simulink model "PassengerCar"  (R2019b)
settings: Solver=ode1  StartTime=0  StopTime=25  FixedStep=1.0000000000000000e-003  RelTol=1e-3
InitFcn:
  | sampleTime = str2double(get_param(bdroot, 'FixedStep'));
undefined symbols (not defined in the file or in its folder): AccPedalPos, BrakePedalPos, BrakeSwitch, DiscIntNeverNeededParam, DYNA4, EngSpd, IgnitionSwitch, InitialGear, InitialSpeed, IntendedEngTrq, LeftIndicator, MainBrakePress, MaxGear, MDL, MinGear, RefAcc, RefLane, RefLatPos, RefPath, RefPathCurv, RefSpd, RefSpdPreview, RefSpdRetrospect, RightIndicator, SteeringWheelAng, SteeringWheelTrq, UserDefinedRefValue, vm_const
libraries: UtilitiesLibrary x31, simulink x18, WheelSystemModules x13, LongitudinalControllerModules x13, LateralControllerModules x7, AnimationBusselectorModules x5, EnvironmentModules x5, BasicEngineControlModules x5, MiscellaneousControlModules x5, Animation3Modules x4, AuxiliariesModules x4, TireModules x4
(part 24 of 39)

== system PassengerCar/Vehicle/WheelSystem/RearLeftWheelSystem/Tire ==
  fromCTRL : Inport
  fromChassis : Inport  Port=2
  fromWheel : Inport  Port=3
  Demux1 : Demux  Outputs=[1 1 1 1 1 1 1]
  Demux2 : Demux  Outputs=[1 1 1 1 1]
  Demux3 : Demux  Outputs=[1 1 1 1 1 1 1]
  Demux4 : Demux  Outputs=[1 1 1]
  Demux5 : Demux  Outputs=[1 1 1]
  DynaComponentInfo : Subsystem  Tag=DynaComponentInfo
      mask init:
      | data= get_param(gcb, 'UserData');
      settings: OpenFcn=DYNA4.ModelHandling.Component.ShowEditComponentInformationDialog(gcb);
      mask Display: disp(['Type = ', data.type, '\nGroup = ', data.group, '\nName = ', data.name])
  InputFromCTRL : Subsystem  Tag=TESIS DYNAware Interface Block  mask{NeedsUpdate=off, SignalInfo=|}
      mask SignalInfo=|
      | {
      |   "Version": "4.6",
      |   "MuxedOutputBusName": "output",
      |   "MuxedInputBusName": "fromCTRL",
      |   "MuxedInputSelected": true,
      |   "MuxedOutputSelected": false,
      |   "SignalData": [
      |     {
      |       "initialValue": "0.0",
      |       "name": "AddRoadElev[m]",
      |       "comment": "",
      |       "minString": "",
      |       "maxString": "",
      |       "width": 1,
      |       "dataType": 0,
      |       "signalType": 0,
      |       "createSignal": false,
      |       "outputName": "AddRoadElev[m]",
      |       "generateSignalAccessBlock": false,
      |       "accessId": "$(parentId).$(blockName).$(outputName)"
      |     },
      |     {
      |       "initialValue": "0.0",
      |       "name": "RoadFrictionScaling[0_2]",
      |       "comment": "",
      |       "minString": "",
      |       "maxString": "",
      |       "width": 1,
      |       "dataType": 0,
      |       "signalType": 0,
      |       "createSignal": false,
      |       "outputName": "RoadFrictionScaling[0_2]",
      |       "generateSignalAccessBlock": false,
      |       "accessId": "$(parentId).$(blockName).$(outputName)"
      |     },
      |     {
      |       "initialValue": "0.0",
      |       "name": "AddLongRoadSlope[-]",
      |       "comment": "",
      |       "minString": "",
      |       "maxString": "",
      |       "width": 1,
      |       "dataType": 0,
      |       "signalType": 0,
      |       "createSignal": false,
      |       "outputName": "AddLongRoadSlope[-]",
      |       "generateSignalAccessBlock": false,
      |       "accessId": "$(parentId).$(blockName).$(outputName)"
      |     },
      |     {
      |       "initialValue": "0.0",
      |       "name": "AddLatRoadSlope[-]",
      |       "comment": "",
      |       "minString": "",
      |       "maxString": "",
      |       "width": 1,
      |       "dataType": 0,
      |       "signalType": 0,
      |       "createSignal": false,
      |       "outputName": "AddLatRoadSlope[-]",
      |       "generateSignalAccessBlock": false,
      |       "accessId": "$(parentId).$(blockName).$(outputName)"
      |     },
      |     {
      |       "initialValue": "0.0",
      |       "name": "LocalRoadSysSwitch[0;1]",
      |       "comment": "",
      |       "minString": "",
      |       "maxString": "",
      |       "width": 1,
      |       "dataType": 0,
      |       "signalType": 0,
      |       "createSignal": false,
      |       "outputName": "LocalRoadSysSwitch[0;1]",
      |       "generateSignalAccessBlock": false,
      |       "accessId": "$(parentId).$(blockName).$(outputName)"
      |     },
      |     {
      |       "initialValue": "0.0",
      |       "name": "RelInflPress[Pa]",
      |       "comment": "",
      |       "minString": "",
      |       "maxString": "",
      |       "width": -1,
      |       "dataType": 0,
      |       "signalType": 0,
      |       "createSignal": false,
      |       "outputName": "RelInflPress[Pa]",
      |       "generateSignalAccessBlock": false,
      |       "accessId": "$(parentId).$(blockName).$(outputName)"
      |     }
      |   ]
      | }
      mask prompts: NeedsUpdate "Specify, if subsystem content needs to be updated"; SignalInfo "Signal Info (json)"
      mask help: DYNA4 Interface Block Version 4.6
      mask init:
      | blockName = get_param(gcbh, 'Name');
      | parentId = DYNA4.ModelHandling.AccessID.getFromHierarchy(gcbh);
      | TD.InterfaceBlock.ModelCallbacks.GenerateContent(gcb);
      settings: DeleteFcn=TD.InterfaceBlock.ModelCallbacks.CloseGUI( gcbh );  NameChangeFcn=TD.InterfaceBlock.ModelCallbacks.BlockRenamedHandler(gcbh);  OpenFcn=TD.InterfaceBlock.ModelCallbacks.OpenGUI( gcbh );  CloseFcn=TD.InterfaceBlock.ModelCallbacks.CloseGUI( gcbh );
      mask Display:
      | image('InterfaceBlock.png','center');
      | port_label('input',1, 'fromCTRL');
      | port_label('output',1, 'AddRoadElev[m]');
      | port_label('output',2, 'RoadFrictionScaling[0_2]');
      | port_label('output',3, 'AddLongRoadSlope[-]');
      | port_label('output',4, 'AddLatRoadSlope[-]');
      | port_label('output',5, 'LocalRoadSysSwitch[0;1]');
      | port_label('output',6, 'RelInflPress[Pa]');
  InputFromChassis : Subsystem  Tag=TESIS DYNAware Interface Block  mask{NeedsUpdate=off, SignalInfo=|}
      mask SignalInfo=|
      | {
      |   "Version": "4.6",
      |   "MuxedOutputBusName": "output",
      |   "MuxedInputBusName": "fromChassis",
      |   "MuxedInputSelected": true,
      |   "MuxedOutputSelected": false,
      |   "SignalData": [
      |     {
      |       "initialValue": "0.0",
      |       "name": "VehicleBody.Pos(WorldSys)[m]",
      |       "comment": "",
      |       "minString": "",
      |       "maxString": "",
      |       "width": 3,
      |       "dataType": 0,
      |       "signalType": 0,
      |       "createSignal": false,
      |       "outputName": "Pos(WorldSys)[m]",
      |       "generateSignalAccessBlock": false,
      |       "accessId": "$(parentId).$(blockName).$(outputName)"
      |     },
      |     {
      |       "initialValue": "0.0",
      |       "name": "VehicleBody.RotMatrix(WorldSys)[-]",
      |       "comment": "",
      |       "minString": "",
      |       "maxString": "",
      |       "width": 9,
      |       "dataType": 0,
      |       "signalType": 0,
      |       "createSignal": false,
      |       "outputName": "RotMatrix(WorldSys)[-]",
      |       "generateSignalAccessBlock": false,
      |       "accessId": "$(parentId).$(blockName).$(outputName)"
      |     },
      |     {
      |       "initialValue": "0.0",
      |       "name": "WheelSystem.WheelRotAxis(VehSys)[-]",
      |       "comment": "",
      |       "minString": "",
      |       "maxString": "",
      |       "width": 3,
      |       "dataType": 0,
      |       "signalType": 0,
      |       "createSignal": false,
      |       "outputName": "WheelRotAxis(VehSys)[-]",
      |       "generateSignalAccessBlock": false,
      |       "accessId": "$(parentId).$(blockName).$(outputName)"
      |     },
      |     {
      |       "initialValue": "0.0",
      |       "name": "WheelSystem.TirePos(VehSys)[m]",
      |       "comment": "",
      |       "minString": "",
      |       "maxString": "",
      |       "width": 3,
      |       "dataType": 0,
      |       "signalType": 0,
      |       "createSignal": false,
      |       "outputName": "TirePos(VehSys)[m]",
      |       "generateSignalAccessBlock": false,
      |       "accessId": "$(parentId).$(blockName).$(outputName)"
      |     },
      |     {
      |       "initialValue": "0.0",
      |       "name": "WheelSystem.TireVel_wrt_WorldSys(VehSys)[m/s]",
      |       "comment": "",
      |       "minString": "",
      |       "maxString": "",
      |       "width": 3,
      |       "dataType": 0,
      |       "signalType": 0,
      |       "createSignal": false,
      |       "outputName": "TireVel_wrt_WorldSys(VehSys)[m/s]",
      |       "generateSignalAccessBlock": false,
      |       "accessId": "$(parentId).$(blockName).$(outputName)"
      |     },
      |     {
      |       "initialValue": "0.0",
      |       "name": "WheelSystem.WheelRotVel_wrt_WorldSys(VehSys)[rad/s]",
      |       "comment": "",
      |       "minString": "",
      |       "maxString": "",
      |       "width": 3,
      |       "dataType": 0,
      |       "signalType": 0,
      |       "createSignal": false,
      |       "outputName": "WheelRotVel_wrt_WorldSys(VehSys)[rad/s]",
      |       "generateSignalAccessBlock": false,
      |       "accessId": "$(parentId).$(blockName).$(outputName)"
      |     }
      |   ]
      | }
      mask prompts: NeedsUpdate "Specify, if subsystem content needs to be updated"; SignalInfo "Signal Info (json)"
      mask help: DYNA4 Interface Block Version 4.6
      mask init:
      | blockName = get_param(gcbh, 'Name');
      | parentId = DYNA4.ModelHandling.AccessID.getFromHierarchy(gcbh);
      | TD.InterfaceBlock.ModelCallbacks.GenerateContent(gcb);
      settings: DeleteFcn=TD.InterfaceBlock.ModelCallbacks.CloseGUI( gcbh );  NameChangeFcn=TD.InterfaceBlock.ModelCallbacks.BlockRenamedHandler(gcbh);  OpenFcn=TD.InterfaceBlock.ModelCallbacks.OpenGUI( gcbh );  CloseFcn=TD.InterfaceBlock.ModelCallbacks.CloseGUI( gcbh );
      mask Display:
      | image('InterfaceBlock.png','center');
      | port_label('input',1, 'fromChassis');
      | port_label('output',1, 'Pos(WorldSys)[m]');
      | port_label('output',2, 'RotMatrix(WorldSys)[-]');
      | port_label('output',3, 'WheelRotAxis(VehSys)[-]');
      | port_label('output',4, 'TirePos(VehSys)[m]');
      | port_label('output',5, 'TireVel_wrt_WorldSys(VehSys)[m/s]');
      | port_label('output',6, 'WheelRotVel_wrt_WorldSys(VehSys)[rad/s]');
  InputFromWheel : Subsystem  Tag=TESIS DYNAware Interface Block  mask{NeedsUpdate=off, SignalInfo=|}
      mask SignalInfo=|
      | {
      |   "Version": "4.6",
      |   "MuxedOutputBusName": "fromWheel",
      |   "MuxedInputBusName": "fromWheel",
      |   "MuxedInputSelected": true,
      |   "MuxedOutputSelected": false,
      |   "SignalData": {
      |     "initialValue": "0.0",
      |     "name": "RotSpd[rad/s]",
      |     "comment": "",
      |     "minString": "",
      |     "maxString": "",
      |     "width": 1,
      |     "dataType": 0,
      |     "signalType": 0,
      |     "createSignal": false,
      |     "outputName": "RotSpd[rad/s]",
      |     "generateSignalAccessBlock": false,
      |     "accessId": "$(parentId).$(blockName).$(outputName)"
      |   }
      | }
      mask prompts: NeedsUpdate "Specify, if subsystem content needs to be updated"; SignalInfo "Signal Info (json)"
      mask help: DYNA4 Interface Block Version 4.6
      mask init:
      | blockName = get_param(gcbh, 'Name');
      | parentId = DYNA4.ModelHandling.AccessID.getFromHierarchy(gcbh);
      | TD.InterfaceBlock.ModelCallbacks.GenerateContent(gcb);
      settings: DeleteFcn=TD.InterfaceBlock.ModelCallbacks.CloseGUI( gcbh );  NameChangeFcn=TD.InterfaceBlock.ModelCallbacks.BlockRenamedHandler(gcbh);  OpenFcn=TD.InterfaceBlock.ModelCallbacks.OpenGUI( gcbh );  CloseFcn=TD.InterfaceBlock.ModelCallbacks.CloseGUI( gcbh );
      mask Display:
      | image('InterfaceBlock.png','center');
      | port_label('input',1, 'fromWheel');
      | port_label('output',1, 'RotSpd[rad/s]');
  TMEasy5 : TireModules/TMEasy5  DATA_NODE=MDL.Vehicle.WheelSystem.RearLeft.Tire.TMEasy5  Enable=MDL.Vehicle.WheelSystem.RearLeft.Tire.TMEasy5.Enable  GeneralConstants=MDL.Vehicle.WheelSystem.RearLeft.Tire.TMEasy5.GeneralConstants  ParameterConstants=MDL.Vehicle.WheelSystem.RearLeft.Tire.TMEasy5.ParameterConstants  AdvancedOptions=MDL.Vehicle.WheelSystem.RearLeft.Tire.TMEasy5.AdvancedOptions  sample_time=-1
  TireOutput : Subsystem  Tag=TESIS DYNAware Interface Block  mask{NeedsUpdate=off, SignalInfo=|}
      mask SignalInfo=|
      | {
      |   "Version": "4.6",
      |   "MuxedOutputBusName": "Tire",
      |   "MuxedInputBusName": "input",
      |   "MuxedInputSelected": false,
      |   "MuxedOutputSelected": true,
      |   "SignalData": [
      |     {
      |       "initialValue": "0.0",
      |       "name": "ContactPointPos_wrt_WheelCenter(WorldSys)[m]",
      |       "comment": "",
      |       "minString": "",
      |       "maxString": "",
      |       "width": 3,
      |       "dataType": 0,
      |       "signalType": 0,
      |       "createSignal": false,
      |       "outputName": "ContactPointPos_wrt_WheelCenter(WorldSys)[m]",
      |       "generateSignalAccessBlock": false,
      |       "accessId": "$(parentId).$(blockName).$(outputName)"
      |     },
      |     {
      |       "initialValue": "0.0",
      |       "name": "CamberAng(ContactSys)[rad]",
      |       "comment": "",
      |       "minString": "",
      |       "maxString": "",
      |       "width": 1,
      |       "dataType": 0,
      |       "signalType": 0,
      |       "createSignal": false,
      |       "outputName": "CamberAng(ContactSys)[rad]",
      |       "generateSignalAccessBlock": false,
      |       "accessId": "$(parentId).$(blockName).$(outputName)"
      |     },
      |     {
      |       "initialValue": "0.0",
      |       "name": "TireDefl[m]",
      |       "comment": "",
      |       "minString": "",
      |       "maxString": "",
      |       "width": 1,
      |       "dataType": 0,
      |       "signalType": 0,
      |       "createSignal": false,
      |       "outputName": "TireDefl[m]",
      |       "generateSignalAccessBlock": false,
      |       "accessId": "$(parentId).$(blockName).$(outputName)"
      |     },
      |     {
      |       "initialValue": "0.0",
      |       "name": "TireDeflSpd[m/s]",
      |       "comment": "",
      |       "minString": "",
      |       "maxString": "",
      |       "width": 1,
      |       "dataType": 0,
      |       "signalType": 0,
      |       "createSignal": false,
      |       "outputName": "TireDeflSpd[m/s]",
      |       "generateSignalAccessBlock": false,
      |       "accessId": "$(parentId).$(blockName).$(outputName)"
      |     },
      |     {
      |       "initialValue": "0.0",
      |       "name": "LongSpd(ContactSys)[m/s]",
      |       "comment": "",
      |       "minString": "",
      |       "maxString": "",
      |       "width": 1,
      |       "dataType": 0,
      |       "signalType": 0,
      |       "createSignal": false,
      |       "outputName": "LongSpd(ContactSys)[m/s]",
      |       "generateSignalAccessBlock": false,
      |       "accessId": "$(parentId).$(blockName).$(outputName)"
      |     },
      |     {
      |       "initialValue": "0.0",
      |       "name": "LatSpd(ContactSys)[m/s]",
      |       "comment": "",
      |       "minString": "",
      |       "maxString": "",
      |       "width": 1,
      |       "dataType": 0,
      |       "signalType": 0,
      |       "createSignal": false,
      |       "outputName": "LatSpd(ContactSys)[m/s]",
      |       "generateSignalAccessBlock": false,
      |       "accessId": "$(parentId).$(blockName).$(outputName)"
      |     },
      |     {
      |       "initialValue": "0.0",
      |       "name": "BoreSpd(ContactSys)[rad/s]",
      |       "comment": "",
      |       "minString": "",
      |       "maxString": "",
      |       "width": 1,
      |       "dataType": 0,
      |       "signalType": 0,
      |       "createSignal": false,
      |       "outputName": "BoreSpd(ContactSys)[rad/s]",
      |       "generateSignalAccessBlock": false,
      |       "accessId": "$(parentId).$(blockName).$(outputName)"
      |     },
      |     {
      |       "initialValue": "0.0",
      |       "name": "LongFrcLeverArm_wrt_WheelRotAxis[m]",
      |       "comment": "",
      |       "minString": "",
      |       "maxString": "",
      |       "width": 1,
      |       "dataType": 0,
      |       "signalType": 0,
      |       "createSignal": false,
      |       "outputName": "LongFrcLeverArm_wrt_WheelRotAxis[m]",
      |       "generateSignalAccessBlock": false,
      |       "accessId": "$(parentId).$(blockName).$(outputName)"
      |     },
      |     {
      |       "initialValue": "0.0",
      |       "name": "LongUnitVector(WorldSys)[-]",
      |       "comment": "",
      |       "minString": "",
      |       "maxString": "",
      |       "width": 3,
      |       "dataType": 0,
      |       "signalType": 0,
      |       "createSignal": false,
      |       "outputName": "LongUnitVector(WorldSys)[-]",
      |       "generateSignalAccessBlock": false,
      |       "accessId": "$(parentId).$(blockName).$(outputName)"
      |     },
      |     {
      |       "initialValue": "0.0",
      |       "name": "LatUnitVector(WorldSys)[-]",
      |       "comment": "",
      |       "minString": "",
      |       "maxString": "",
      |       "width": 3,
      |       "dataType": 0,
      |       "signalType": 0,
      |       "createSignal": false,
      |       "outputName": "LatUnitVector(WorldSys)[-]",
      |       "generateSignalAccessBlock": false,
      |       "accessId": "$(parentId).$(blockName).$(outputName)"
      |     },
      |     {
      |       "initialValue": "0.0",
      |       "name": "RoadNormalVector(WorldSys)[-]",
      |       "comment": "",
      |       "minString": "",
      |       "maxString": "",
      |       "width": 3,
      |       "dataType": 0,
      |       "signalType": 0,
      |       "createSignal": false,
      |       "outputName": "RoadNormalVector(WorldSys)[-]",
      |       "generateSignalAccessBlock": false,
      |       "accessId": "$(parentId).$(blockName).$(outputName)"
      |     },
      |     {
      |       "initialValue": "0.0",
      |       "name": "RoadType[-]",
      |       "comment": "",
      |       "minString": "",
      |       "maxString": "",
      |       "width": 1,
      |       "dataType": 0,
      |       "signalType": 0,
      |       "createSignal": false,
      |       "outputName": "RoadType[-]",
      |       "generateSignalAccessBlock": false,
      |       "accessId": "$(parentId).$(blockName).$(outputName)"
      |     },
      |     {
      |       "initialValue": "0.0",
      |       "name": "RoadFrictionScalingCoeff[-]",
      |       "comment": "",
      |       "minString": "",
      |       "maxString": "",
      |       "width": 1,
      |       "dataType": 0,
      |       "signalType": 0,
      |       "createSignal": false,
      |       "outputName": "RoadFrictionScalingCoeff[-]",
      |       "generateSignalAccessBlock": false,
      |       "accessId": "$(parentId).$(blockName).$(outputName)"
      |     },
      |     {
      |       "initialValue": "0.0",
      |       "name": "ContactPointPos(WorldSys)[m]",
      |       "comment": "",
      |       "minString": "",
      |       "maxString": "",
      |       "width": 3,
      |       "dataType": 0,
      |       "signalType": 0,
      |       "createSignal": false,
      |       "outputName": "ContactPointPos(WorldSys)[m]",
      |       "generateSignalAccessBlock": false,
      |       "accessId": "$(parentId).$(blockName).$(outputName)"
      |     },
      |     {
      |       "initialValue": "0.0",
      |       "name": "WheelCenterFrc(VehSys)[N]",
      |       "comment": "",
      |       "minString": "",
      |       "maxString": "",
      |       "width": 3,
      |       "dataType": 0,
      |       "signalType": 0,
      |       "createSignal": false,
      |       "outputName": "WheelCenterFrc(VehSys)[N]",
      |       "generateSignalAccessBlock": false,
      |       "accessId": "$(parentId).$(blockName).$(outputName)"
      |     },
      |     {
      |       "initialValue": "0.0",
      |       "name": "WheelCenterTrq(VehSys)[Nm]",
      |       "comment": "",
      |       "minString": "",
      |       "maxString": "",
      |       "width": 3,
      |       "dataType": 0,
      |       "signalType": 0,
      |       "createSignal": false,
      |       "outputName": "WheelCenterTrq(VehSys)[Nm]",
      |       "generateSignalAccessBlock": false,
      |       "accessId": "$(parentId).$(blockName).$(outputName)"
      |     },
      |     {
      |       "initialValue": "0.0",
      |       "name": "CircumferentialTrq_wrt_WheelRotAxis[Nm]",
      |       "comment": "",
      |       "minString": "",
      |       "maxString": "",
      |       "width": 1,
      |       "dataType": 0,
      |       "signalType": 0,
      |       "createSignal": false,
      |       "outputName": "CircumferentialTrq_wrt_WheelRotAxis[Nm]",
      |       "generateSignalAccessBlock": false,
      |       "accessId": "$(parentId).$(blockName).$(outputName)"
      |     },
      |     {
      |       "initialValue": "0.0",
      |       "name": "MaxRollResistTrq[Nm]",
      |       "comment": "",
      |       "minString": "",
      |       "maxString": "",
      |       "width": 1,
      |       "dataType": 0,
      |       "signalType": 0,
      |       "createSignal": false,
      |       "outputName": "MaxRollResistTrq[Nm]",
      |       "generateSignalAccessBlock": false,
      |       "accessId": "$(parentId).$(blockName).$(outputName)"
      |     },
      |     {
      |       "initialValue": "0.0",
      |       "name": "LatDefl(ContactSys)[m]",
      |       "comment": "",
      |       "minString": "",
      |       "maxString": "",
      |       "width": 1,
      |       "dataType": 0,
      |       "signalType": 0,
      |       "createSignal": false,
      |       "outputName": "LatDefl(ContactSys)[m]",
      |       "generateSignalAccessBlock": false,
      |       "accessId": "$(parentId).$(blockName).$(outputName)"
      |     },
      |     {
      |       "initialValue": "0.0",
      |       "name": "VertStiff[N/m]",
      |       "comment": "",
      |       "minString": "",
      |       "maxString": "",
      |       "width": 1,
      |       "dataType": 0,
      |       "signalType": 0,
      |       "createSignal": false,
      |       "outputName": "VertStiff[N/m]",
      |       "generateSignalAccessBlock": false,
      |       "accessId": "$(parentId).$(blockName).$(outputName)"
      |     },
      |     {
      |       "initialValue": "0.0",
      |       "name": "UnloadedRadius[m]",
      |       "comment": "",
      |       "minString": "",
      |       "maxString": "",
      |       "width": 1,
      |       "dataType": 0,
      |       "signalType": 0,
      |       "createSignal": false,
      |       "outputName": "UnloadedRadius[m]",
      |       "generateSignalAccessBlock": false,
      |       "accessId": "$(parentId).$(blockName).$(outputName)"
      |     },
      |     {
      |       "initialValue": "0.0",
      |       "name": "RimRadius[m]",
      |       "comment": "",
      |       "minString": "",
      |       "maxString": "",
      |       "width": 1,
      |       "dataType": 0,
      |       "signalType": 0,
      |       "createSignal": false,
      |       "outputName": "RimRadius[m]",
      |       "generateSignalAccessBlock": false,
      |       "accessId": "$(parentId).$(blockName).$(outputName)"
      |     },
      |     {
      |       "initialValue": "0.0",
      |       "name": "Width[m]",
      |       "comment": "",
      |       "minString": "",
      |       "maxString": "",
      |       "width": 1,
      |       "dataType": 0,
      |       "signalType": 0,
      |       "createSignal": false,
      |       "outputName": "Width[m]",
      |       "generateSignalAccessBlock": false,
      |       "accessId": "$(parentId).$(blockName).$(outputName)"
      |     },
      |     {
      |       "initialValue": "0.0",
      |       "name": "ContactPointFrc(ContactSys)[N]",
      |       "comment": "",
      |       "minString": "",
      |       "maxString": "",
      |       "width": 3,
      |       "dataType": 0,
      |       "signalType": 0,
      |       "createSignal": false,
      |       "outputName": "ContactPointFrc(ContactSys)[N]",
      |       "generateSignalAccessBlock": false,
      |       "accessId": "$(parentId).$(blockName).$(outputName)"
      |     },
      |     {
      |       "initialValue": "0.0",
      |       "name": "CorneringStiff[N]",
      |       "comment": "",
      |       "minString": "",
      |       "maxString": "",
      |       "width": 1,
      |       "dataType": 0,
      |       "signalType": 0,
      |       "createSignal": false,
      |       "outputName": "CorneringStiff[N]",
      |       "generateSignalAccessBlock": false,
      |       "accessId": "$(parentId).$(blockName).$(outputName)"
      |     },
      |     {
      |       "initialValue": "0.0",
      |       "name": "DynamicRadius[m]",
      |       "comment": "",
      |       "minString": "",
      |       "maxString": "",
      |       "width": 1,
      |       "dataType": 0,
      |       "signalType": 0,
      |       "createSignal": false,
      |       "outputName": "DynamicRadius[m]",
      |       "generateSignalAccessBlock": false,
      |       "accessId": "$(parentId).$(blockName).$(outputName)"
      |     },
      |     {
      |       "initialValue": "0.0",
      |       "name": "Stabilization.DerivativeOfLongFrc_wrt_LongSpd(ContactSys)[N/(m/s)]",
      |       "comment": "",
      |       "minString": "",
      |       "maxString": "",
      |       "width": 1,
      |       "dataType": 0,
      |       "signalType": 0,
      |       "createSignal": false,
      |       "outputName": "Stabilization.DerivativeOfLongFrc_wrt_LongSpd(ContactSys)[N/(m/s)]",
      |       "generateSignalAccessBlock": false,
      |       "accessId": "$(parentId).$(blockName).$(outputName)"
      |     },
      |     {
      |       "initialValue": "0.0",
      |       "name": "Stabilization.DerivativeOfLongTrq_wrt_LongSpd(ContactSys)[Nm/(m/s)]",
      |       "comment": "",
      |       "minString": "",
      |       "maxString": "",
      |       "width": 1,
      |       "dataType": 0,
      |       "signalType": 0,
      |       "createSignal": false,
      |       "outputName": "Stabilization.DerivativeOfLongTrq_wrt_LongSpd(ContactSys)[Nm/(m/s)]",
      |       "generateSignalAccessBlock": false,
      |       "accessId": "$(parentId).$(blockName).$(outputName)"
      |     },
      |     {
      |       "initialValue": "0.0",
      |       "name": "Stabilization.DerivativeOfLatFrc_wrt_LatSpd(ContactSys)[N/(m/s)]",
      |       "comment": "",
      |       "minString": "",
      |       "maxString": "",
      |       "width": 1,
      |       "dataType": 0,
      |       "signalType": 0,
      |       "createSignal": false,
      |       "outputName": "Stabilization.DerivativeOfLatFrc_wrt_LatSpd(ContactSys)[N/(m/s)]",
      |       "generateSignalAccessBlock": false,
      |       "accessId": "$(parentId).$(blockName).$(outputName)"
      |     },
      |     {
      |       "initialValue": "0.0",
      |       "name": "Stabilization.DerivativeOfLatTrq_wrt_LatSpd(ContactSys)[Nm/(m/s)]",
      |       "comment": "",
      |       "minString": "",
      |       "maxString": "",
      |       "width": 1,
      |       "dataType": 0,
      |       "signalType": 0,
      |       "createSignal": false,
      |       "outputName": "Stabilization.DerivativeOfLatTrq_wrt_LatSpd(ContactSys)[Nm/(m/s)]",
      |       "generateSignalAccessBlock": false,
      |       "accessId": "$(parentId).$(blockName).$(outputName)"
      |     },
      |     {
      |       "initialValue": "0.0",
      |       "name": "Stabilization.DerivativeOfBoreTrq_wrt_BoreSpd(ContactSys)[Nm/(rad/s)]",
      |       "comment": "",
      |       "minString": "",
      |       "maxString": "",
      |       "width": 1,
      |       "dataType": 0,
      |       "signalType": 0,
      |       "createSignal": false,
      |       "outputName": "Stabilization.DerivativeOfBoreTrq_wrt_BoreSpd(ContactSys)[Nm/(rad/s)]",
      |       "generateSignalAccessBlock": false,
      |       "accessId": "$(parentId).$(blockName).$(outputName)"
      |     },
      |     {
      |       "initialValue": "0.0",
      |       "name": "SelfAligningTrq[Nm]",
      |       "comment": "",
      |       "minString": "",
      |       "maxString": "",
      |       "width": 1,
      |       "dataType": 0,
      |       "signalType": 0,
      |       "createSignal": false,
      |       "outputName": "SelfAligningTrq[Nm]",
      |       "generateSignalAccessBlock": false,
      |       "accessId": "$(parentId).$(blockName).$(outputName)"
      |     },
      |     {
      |       "initialValue": "0.0",
      |       "name": "RollResistTrq[Nm]",
      |       "comment": "",
      |       "minString": "",
      |       "maxString": "",
      |       "width": 1,
      |       "dataType": 0,
      |       "signalType": 0,
      |       "createSignal": false,
      |       "outputName": "RollResistTrq[Nm]",
      |       "generateSignalAccessBlock": false,
      |       "accessId": "$(parentId).$(blockName).$(outputName)"
      |     },
      |     {
      |       "initialValue": "0.0",
      |       "name": "TippingTrq[Nm]",
      |       "comment": "",
      |       "minString": "",
      |       "maxString": "",
      |       "width": 1,
      |       "dataType": 0,
      |       "signalType": 0,
      |       "createSignal": false,
      |       "outputName": "TippingTrq[Nm]",
      |       "generateSignalAccessBlock": false,
      |       "accessId": "$(parentId).$(blockName).$(outputName)"
      |     },
      |     {
      |       "initialValue": "0.0",
      |       "name": "BoreTrq[Nm]",
      |       "comment": "",
      |       "minString": "",
      |       "maxString": "",
      |       "width": 1,
      |       "dataType": 0,
      |       "signalType": 0,
      |       "createSignal": false,
      |       "outputName": "BoreTrq[Nm]",
      |       "generateSignalAccessBlock": false,
      |       "accessId": "$(parentId).$(blockName).$(outputName)"
      |     },
      |     {
      |       "initialValue": "0.0",
      |       "name": "NormalizedLongSlip[-]",
      |       "comment": "",
      |       "minString": "",
      |       "maxString": "",
      |       "width": 1,
      |       "dataType": 0,
      |       "signalType": 0,
      |       "createSignal": false,
      |       "outputName": "NormalizedLongSlip[-]",
      |       "generateSignalAccessBlock": false,
      |       "accessId": "$(parentId).$(blockName).$(outputName)"
      |     },
      |     {
      |       "initialValue": "0.0",
      |       "name": "NormalizedLatSlip[-]",
      |       "comment": "",
      |       "minString": "",
      |       "maxString": "",
      |       "width": 1,
      |       "dataType": 0,
      |       "signalType": 0,
      |       "createSignal": false,
      |       "outputName": "NormalizedLatSlip[-]",
      |       "generateSignalAccessBlock": false,
      |       "accessId": "$(parentId).$(blockName).$(outputName)"
      |     },
      |     {
      |       "initialValue": "0.0",
      |       "name": "LongSlip[-]",
      |       "comment": "",
      |       "minString": "",
      |       "maxString": "",
      |       "width": 1,
      |       "dataType": 0,
      |       "signalType": 0,
      |       "createSignal": false,
      |       "outputName": "LongSlip[-]",
      |       "generateSignalAccessBlock": false,
      |       "accessId": "$(parentId).$(blockName).$(outputName)"
      |     },
      |     {
      |       "initialValue": "0.0",
      |       "name": "LatSlip[-]",
      |       "comment": "",
      |       "minString": "",
      |       "maxString": "",
      |       "width": 1,
      |       "dataType": 0,
      |       "signalType": 0,
      |       "createSignal": false,
      |       "outputName": "LatSlip[-]",
      |       "generateSignalAccessBlock": false,
      |       "accessId": "$(parentId).$(blockName).$(outputName)"
      |     },
      |     {
      |       "initialValue": "0.0",
      |       "name": "BoreSlip[-]",
      |       "comment": "",
      |       "minString": "",
      |       "maxString": "",
      |       "width": 1,
      |       "dataType": 0,
      |       "signalType": 0,
      |       "createSignal": false,
      |       "outputName": "BoreSlip[-]",
      |       "generateSignalAccessBlock": false,
      |       "accessId": "$(parentId).$(blockName).$(outputName)"
      |     },
      |     {
      |       "initialValue": "0.0",
      |       "name": "CombinedSlip[-]",
      |       "comment": "",
      |       "minString": "",
      |       "maxString": "",
      |       "width": 1,
      |       "dataType": 0,
      |       "signalType": 0,
      |       "createSignal": false,
      |       "outputName": "CombinedSlip[-]",
      |       "generateSignalAccessBlock": false,
      |       "accessId": "$(parentId).$(blockName).$(outputName)"
      |     },
      |     {
      |       "initialValue": "0.0",
      |       "name": "GeneralizedSlip[-]",
      |       "comment": "",
      |       "minString": "",
      |       "maxString": "",
      |       "width": 1,
      |       "dataType": 0,
      |       "signalType": 0,
      |       "createSignal": false,
      |       "outputName": "GeneralizedSlip[-]",
      |       "generateSignalAccessBlock": false,
      |       "accessId": "$(parentId).$(blockName).$(outputName)"
      |     },
      |     {
      |       "initialValue": "0.0",
      |       "name": "GradientOfCombinedFrcAtNoSlip[N/-]",
      |       "comment": "",
      |       "minString": "",
      |       "maxString": "",
      |       "width": 1,
      |       "dataType": 0,
      |       "signalType": 0,
      |       "createSignal": false,
      |       "outputName": "GradientOfCombinedFrcAtNoSlip[N/-]",
      |       "generateSignalAccessBlock": false,
      |       "accessId": "$(parentId).$(blockName).$(outputName)"
      |     },
      |     {
      |       "initialValue": "0.0",
      |       "name": "CombinedMaxFrc[N]",
      |       "comment": "",
      |       "minString": "",
      |       "maxString": "",
      |       "width": 1,
      |       "dataType": 0,
      |       "signalType": 0,
      |       "createSignal": false,
      |       "outputName": "CombinedMaxFrc[N]",
      |       "generateSignalAccessBlock": false,
      |       "accessId": "$(parentId).$(blockName).$(outputName)"
      |     },
      |     {
      |       "initialValue": "0.0",
      |       "name": "CombinedMaxSlipAtCombinedMaxFrc[-]",
      |       "comment": "",
      |       "minString": "",
      |       "maxString": "",
      |       "width": 1,
      |       "dataType": 0,
      |       "signalType": 0,
      |       "createSignal": false,
      |       "outputName": "CombinedMaxSlipAtCombinedMaxFrc[-]",
      |       "generateSignalAccessBlock": false,
      |       "accessId": "$(parentId).$(blockName).$(outputName)"
      |     },
      |     {
      |       "initialValue": "0.0",
      |       "name": "CombinedSlideFrc[N]",
      |       "comment": "",
      |       "minString": "",
      |       "maxString": "",
      |       "width": 1,
      |       "dataType": 0,
      |       "signalType": 0,
      |       "createSignal": false,
      |       "outputName": "CombinedSlideFrc[N]",
      |       "generateSignalAccessBlock": false,
      |       "accessId": "$(parentId).$(blockName).$(outputName)"
      |     },
      |     {
      |       "initialValue": "0.0",
      |       "name": "CombinedSlipAtCombinedSlideFrc[-]",
      |       "comment": "",
      |       "minString": "",
      |       "maxString": "",
      |       "width": 1,
      |       "dataType": 0,
      |       "signalType": 0,
      |       "createSignal": false,
      |       "outputName": "CombinedSlipAtCombinedSlideFrc[-]",
      |       "generateSignalAccessBlock": false,
      |       "accessId": "$(parentId).$(blockName).$(outputName)"
      |     },
      |     {
      |       "initialValue": "0.0",
      |       "name": "CombinedForce[N]",
      |       "comment": "",
      |       "minString": "",
      |       "maxString": "",
      |       "width": 1,
      |       "dataType": 0,
      |       "signalType": 0,
      |       "createSignal": false,
      |       "outputName": "CombinedForce[N]",
      |       "generateSignalAccessBlock": false,
      |       "accessId": "$(parentId).$(blockName).$(outputName)"
      |     },
      |     {
      |       "initialValue": "0.0",
      |       "name": "DerivativeOfCombinedFrc_wrt_CombinedSlip[N/-]",
      |       "comment": "",
      |       "minString": "",
      |       "maxString": "",
      |       "width": 1,
      |       "dataType": 0,
      |       "signalType": 0,
      |       "createSignal": false,
      |       "outputName": "DerivativeOfCombinedFrc_wrt_CombinedSlip[N/-]",
      |       "generateSignalAccessBlock": false,
      |       "accessId": "$(parentId).$(blockName).$(outputName)"
      |     },
      |     {
      |       "initialValue": "0.0",
      |       "name": "BoreRadius[m]",
      |       "comment": "",
      |       "minString": "",
      |       "maxString": "",
      |       "width": 1,
      |       "dataType": 0,
      |       "signalType": 0,
      |       "createSignal": false,
      |       "outputName": "BoreRadius[m]",
      |       "generateSignalAccessBlock": false,
      |       "accessId": "$(parentId).$(blockName).$(outputName)"
      |     },
      |     {
      |       "initialValue": "0.0",
      |       "name": "TireRotSpd[rad/s]",
      |       "comment": "",
      |       "minString": "",
      |       "maxString": "",
      |       "width": 1,
      |       "dataType": 0,
      |       "signalType": 0,
      |       "createSignal": false,
      |       "outputName": "TireRotSpd[rad/s]",
      |       "generateSignalAccessBlock": false,
      |       "accessId": "$(parentId).$(blockName).$(outputName)"
      |     },
      |     {
      |       "initialValue": "0.0",
      |       "name": "CamberFrc[N]",
      |       "comment": "",
      |       "minString": "",
      |       "maxString": "",
      |       "width": 1,
      |       "dataType": 0,
      |       "signalType": 0,
      |       "createSignal": false,
      |       "outputName": "CamberFrc[N]",
      |       "generateSignalAccessBlock": false,
      |       "accessId": "$(parentId).$(blockName).$(outputName)"
      |     },
      |     {
      |       "initialValue": "0.0",
      |       "name": "LongRelaxationTime[s]",
      |       "comment": "",
      |       "minString": "",
      |       "maxString": "",
      |       "width": 1,
      |       "dataType": 0,
      |       "signalType": 0,
      |       "createSignal": false,
      |       "outputName": "LongRelaxationTime[s]",
      |       "generateSignalAccessBlock": false,
      |       "accessId": "$(parentId).$(blockName).$(outputName)"
      |     },
      |     {
      |       "initialValue": "0.0",
      |       "name": "LatRelaxationTime[s]",
      |       "comment": "",
      |       "minString": "",
      |       "maxString": "",
      |       "width": 1,
      |       "dataType": 0,
      |       "signalType": 0,
      |       "createSignal": false,
      |       "outputName": "LatRelaxationTime[s]",
      |       "generateSignalAccessBlock": false,
      |       "accessId": "$(parentId).$(blockName).$(outputName)"
      |     },
      |     {
      |       "initialValue": "0.0",
      |       "name": "TorsionalRelaxationTime[s]",
      |       "comment": "",
      |       "minString": "",
      |       "maxString": "",
      |       "width": 1,
      |       "dataType": 0,
      |       "signalType": 0,
      |       "createSignal": false,
      |       "outputName": "TorsionalRelaxationTime[s]",
      |       "generateSignalAccessBlock": false,
      |       "accessId": "$(parentId).$(blockName).$(outputName)"
      |     },
      |     {
      |       "initialValue": "0.0",
      |       "name": "LongRelaxationLength[m]",
      |       "comment": "",
      |       "minString": "",
      |       "maxString": "",
      |       "width": 1,
      |       "dataType": 0,
      |       "signalType": 0,
      |       "createSignal": false,
      |       "outputName": "LongRelaxationLength[m]",
      |       "generateSignalAccessBlock": false,
      |       "accessId": "$(parentId).$(blockName).$(outputName)"
      |     },
      |     {
      |       "initialValue": "0.0",
      |       "name": "LatRelaxationLength[m]",
      |       "comment": "",
      |       "minString": "",
      |       "maxString": "",
      |       "width": 1,
      |       "dataType": 0,
      |       "signalType": 0,
      |       "createSignal": false,
      |       "outputName": "LatRelaxationLength[m]",
      |       "generateSignalAccessBlock": false,
      |       "accessId": "$(parentId).$(blockName).$(outputName)"
      |     },
      |     {
      |       "initialValue": "0.0",
      |       "name": "TorsionalRelaxationAngle[rad]",
      |       "comment": "",
      |       "minString": "",
      |       "maxString": "",
      |       "width": 1,
      |       "dataType": 0,
      |       "signalType": 0,
      |       "createSignal": false,
      |       "outputName": "TorsionalRelaxationAngle[rad]",
      |       "generateSignalAccessBlock": false,
      |       "accessId": "$(parentId).$(blockName).$(outputName)"
      |     },
      |     {
      |       "initialValue": "0.0",
      |       "name": "ContactPointTrq(ContactSys)[Nm]",
      |       "comment": "",
      |       "minString": "",
      |       "maxString": "",
      |       "width": 3,
      |       "dataType": 0,
      |       "signalType": 0,
      |       "createSignal": false,
      |       "outputName": "ContactPointTrq(ContactSys)[Nm]",
      |       "generateSignalAccessBlock": false,
      |       "accessId": "$(parentId).$(blockName).$(outputName)"
      |     },
      |     {
      |       "initialValue": "0.0",
      |       "name": "ContactPatchLength[m]",
      |       "comment": "",
      |       "minString": "",
      |       "maxString": "",
      |       "width": 1,
      |       "dataType": 0,
      |       "signalType": 0,
      |       "createSignal": false,
      |       "outputName": "ContactPatchLength[m]",
      |       "generateSignalAccessBlock": false,
      |       "accessId": "$(parentId).$(blockName).$(outputName)"
      |     },
      |     {
      |       "initialValue": "0.0",
      |       "name": "ContactPatchWidth[m]",
      |       "comment": "",
      |       "minString": "",
      |       "maxString": "",
      |       "width": 1,
      |       "dataType": 0,
      |       "signalType": 0,
      |       "createSignal": false,
      |       "outputName": "ContactPatchWidth[m]",
      |       "generateSignalAccessBlock": false,
      |       "accessId": "$(parentId).$(blockName).$(outputName)"
      |     },
      |     {
      |       "initialValue": "0.0",
      |       "name": "LocalContactPoints(WorldSys)[m]",
      |       "comment": "",
      |       "minString": "",
      |       "maxString": "",
      |       "width": 12,
      |       "dataType": 0,
      |       "signalType": 0,
      |       "createSignal": false,
      |       "outputName": "LocalContactPoints(WorldSys)[m]",
      |       "generateSignalAccessBlock": false,
      |       "accessId": "$(parentId).$(blockName).$(outputName)"
      |     },
      |     {
      |       "initialValue": "0.0",
      |       "name": "NumberOfLocalContactPoints[-]",
      |       "comment": "",
      |       "minString": "",
      |       "maxString": "",
      |       "width": 1,
      |       "dataType": 0,
      |       "signalType": 0,
      |       "createSignal": false,
      |       "outputName": "NumberOfLocalContactPoints[-]",
      |       "generateSignalAccessBlock": false,
      |       "accessId": "$(parentId).$(blockName).$(outputName)"
      |     }
      |   ]
      | }
      mask prompts: NeedsUpdate "Specify, if subsystem content needs to be updated"; SignalInfo "Signal Info (json)"
      mask help: DYNA4 Interface Block Version 4.6
      mask init:
      | blockName = get_param(gcbh, 'Name');
      | parentId = DYNA4.ModelHandling.AccessID.getFromHierarchy(gcbh);
      | TD.InterfaceBlock.ModelCallbacks.GenerateContent(gcb);
      settings: DeleteFcn=TD.InterfaceBlock.ModelCallbacks.CloseGUI( gcbh );  NameChangeFcn=TD.InterfaceBlock.ModelCallbacks.BlockRenamedHandler(gcbh);  OpenFcn=TD.InterfaceBlock.ModelCallbacks.OpenGUI( gcbh );  CloseFcn=TD.InterfaceBlock.ModelCallbacks.CloseGUI( gcbh );
      mask Display:
      | image('InterfaceBlock.png','center');
      | port_label('input',1, 'ContactPointPos_wrt_WheelCenter(WorldSys)[m]');
      | port_label('input',2, 'CamberAng(ContactSys)[rad]');
      | port_label('input',3, 'TireDefl[m]');
      | port_label('input',4, 'TireDeflSpd[m/s]');
      | port_label('input',5, 'LongSpd(ContactSys)[m/s]');
      | port_label('input',6, 'LatSpd(ContactSys)[m/s]');
      | port_label('input',7, 'BoreSpd(ContactSys)[rad/s]');
      | port_label('input',8, 'LongFrcLeverArm_wrt_WheelRotAxis[m]');
      | port_label('input',9, 'LongUnitVector(WorldSys)[-]');
      | port_label('input',10, 'LatUnitVector(WorldSys)[-]');
      | port_label('input',11, 'RoadNormalVector(WorldSys)[-]');
      | port_label('input',12, 'RoadType[-]');
      | port_label('input',13, 'RoadFrictionScalingCoeff[-]');
      | port_label('input',14, 'ContactPointPos(WorldSys)[m]');
      | port_label('input',15, 'WheelCenterFrc(VehSys)[N]');
      | port_label('input',16, 'WheelCenterTrq(VehSys)[Nm]');
      | port_label('input',17, 'CircumferentialTrq_wrt_WheelRotAxis[Nm]');
      | port_label('input',18, 'MaxRollResistTrq[Nm]');
      | port_label('input',19, 'LatDefl(ContactSys)[m]');
      | port_label('input',20, 'VertStiff[N/m]');
      | port_label('input',21, 'UnloadedRadius[m]');
      | port_label('input',22, 'RimRadius[m]');
      | port_label('input',23, 'Width[m]');
      | port_label('input',24, 'ContactPointFrc(ContactSys)[N]');
      | port_label('input',25, 'CorneringStiff[N]');
      | port_label('input',26, 'DynamicRadius[m]');
      | port_label('input',27, 'Stabilization.DerivativeOfLongFrc_wrt_LongSpd(ContactSys)[N/(m/s)]');
      | port_label('input',28, 'Stabilization.DerivativeOfLongTrq_wrt_LongSpd(ContactSys)[Nm/(m/s)]');
      | port_label('input',29, 'Stabilization.DerivativeOfLatFrc_wrt_LatSpd(ContactSys)[N/(m/s)]');
      | port_label('input',30, 'Stabilization.DerivativeOfLatTrq_wrt_LatSpd(ContactSys)[Nm/(m/s)]');
      | port_label('input',31, 'Stabilization.DerivativeOfBoreTrq_wrt_BoreSpd(ContactSys)[Nm/(rad/s)]');
      | port_label('input',32, 'SelfAligningTrq[Nm]');
      | port_label('input',33, 'RollResistTrq[Nm]');
      | port_label('input',34, 'TippingTrq[Nm]');
      | port_label('input',35, 'BoreTrq[Nm]');
      | port_label('input',36, 'NormalizedLongSlip[-]');
      | port_label('input',37, 'NormalizedLatSlip[-]');
      | port_label('input',38, 'LongSlip[-]');
      | port_label('input',39, 'LatSlip[-]');
      | port_label('input',40, 'BoreSlip[-]');
      | port_label('input',41, 'CombinedSlip[-]');
      | port_label('input',42, 'GeneralizedSlip[-]');
      | port_label('input',43, 'GradientOfCombinedFrcAtNoSlip[N/-]');
      | port_label('input',44, 'CombinedMaxFrc[N]');
      | port_label('input',45, 'CombinedMaxSlipAtCombinedMaxFrc[-]');
      | port_label('input',46, 'CombinedSlideFrc[N]');
      | port_label('input',47, 'CombinedSlipAtCombinedSlideFrc[-]');
      | port_label('input',48, 'CombinedForce[N]');
      | port_label('input',49, 'DerivativeOfCombinedFrc_wrt_CombinedSlip[N/-]');
      | port_label('input',50, 'BoreRadius[m]');
      | port_label('input',51, 'TireRotSpd[rad/s]');
      | port_label('input',52, 'CamberFrc[N]');
      | port_label('input',53, 'LongRelaxationTime[s]');
      | port_label('input',54, 'LatRelaxationTime[s]');
      | port_label('input',55, 'TorsionalRelaxationTime[s]');
      | port_label('input',56, 'LongRelaxationLength[m]');
      | port_label('input',57, 'LatRelaxationLength[m]');
      | port_label('input',58, 'TorsionalRelaxationAngle[rad]');
      | port_label('input',59, 'ContactPointTrq(ContactSys)[Nm]');
      | port_label('input',60, 'ContactPatchLength[m]');
      | port_label('input',61, 'ContactPatchWidth[m]');
      | port_label('input',62, 'LocalContactPoints(WorldSys)[m]');
      | port_label('input',63, 'NumberOfLocalContactPoints[-]');
      | port_label('output',1, 'Tire');
  TraceMarker : UtilitiesLibrary/DYNA4 Trace Marker  Tag=DYNA4_TRACE_MARKER  SettingType=Standard  PrefixModelBlockID=on  PrefixRootSignalName=off  NamePattern='$(modelBlockID).$(rootSignalName)'
  Tire : Outport  VectorParamsAs1DForOutWhenUnconnected=off
  wires:
  InputFromCTRL/6(RelInflPress[Pa]___UNIQUE_1) -> TMEasy5/13
  fromWheel/1 -> InputFromWheel/1(fromWheel)
  fromCTRL/1 -> InputFromCTRL/1(fromCTRL)
  fromChassis/1 -> InputFromChassis/1(fromChassis)
  Demux2/5 -> TireOutput/31(DerivativeOfBoreTrq_wrt_BoreSpd(ContactSys)[Nm/(rad/s)]___UNIQUE_1)
  Demux2/4 -> TireOutput/30(DerivativeOfLatTrq_wrt_LatSpd(ContactSys)[Nm/(m/s)]___UNIQUE_1)
  Demux2/3 -> TireOutput/29(DerivativeOfLatFrc_wrt_LatSpd(ContactSys)[N/(m/s)]___UNIQUE_1)
  Demux2/2 -> TireOutput/28(DerivativeOfLongTrq_wrt_LongSpd(ContactSys)[Nm/(m/s)]___UNIQUE_1)
  Demux2/1 -> TireOutput/27(DerivativeOfLongFrc_wrt_LongSpd(ContactSys)[N/(m/s)]___UNIQUE_1)
  TireOutput/1(Tire___UNIQUE_1) -> TraceMarker/1, Tire/1
  InputFromWheel/1(RotSpd[rad/s]___UNIQUE_1) -> TMEasy5/1
  Demux1/1 -> TireOutput/36(NormalizedLongSlip[-]___UNIQUE_1)
  Demux1/2 -> TireOutput/37(NormalizedLatSlip[-]___UNIQUE_1)
  Demux1/3 -> TireOutput/38(LongSlip[-]___UNIQUE_1)
  Demux1/4 -> TireOutput/39(LatSlip[-]___UNIQUE_1)
  Demux1/5 -> TireOutput/40(BoreSlip[-]___UNIQUE_1)
  Demux1/6 -> TireOutput/41(CombinedSlip[-]___UNIQUE_1)
  Demux1/7 -> TireOutput/42(GeneralizedSlip[-]___UNIQUE_1)
  Demux3/1 -> TireOutput/43(GradientOfCombinedFrcAtNoSlip[N/-]___UNIQUE_1)
  Demux3/2 -> TireOutput/44(CombinedMaxFrc[N]___UNIQUE_1)
  Demux3/3 -> TireOutput/45(CombinedMaxSlipAtCombinedMaxFrc[-]___UNIQUE_1)
  Demux3/4 -> TireOutput/46(CombinedSlideFrc[N]___UNIQUE_1)
  Demux3/5 -> TireOutput/47(CombinedSlipAtCombinedSlideFrc[-]___UNIQUE_1)
  Demux3/6 -> TireOutput/48(CombinedForce[N]___UNIQUE_1)
  Demux3/7 -> TireOutput/49(DerivativeOfCombinedFrc_wrt_CombinedSlip[N/-]___UNIQUE_1)
  InputFromChassis/1(Pos(WorldSys)[m]___UNIQUE_1) -> TMEasy5/2
  InputFromChassis/2(RotMatrix(WorldSys)[-]___UNIQUE_1) -> TMEasy5/3
  InputFromChassis/3(WheelRotAxis(VehSys)[-]___UNIQUE_1) -> TMEasy5/4
  InputFromChassis/4(TirePos(VehSys)[m]___UNIQUE_1) -> TMEasy5/5
  InputFromChassis/5(TireVel_wrt_WorldSys(VehSys)[m/s]___UNIQUE_1) -> TMEasy5/6
  InputFromChassis/6(WheelRotVel_wrt_WorldSys(VehSys)[rad/s]___UNIQUE_1) -> TMEasy5/7
  InputFromCTRL/1(AddRoadElev[m]___UNIQUE_1) -> TMEasy5/8
  InputFromCTRL/2(RoadFrictionScaling[0_2]___UNIQUE_1) -> TMEasy5/9
  InputFromCTRL/3(AddLongRoadSlope[-]___UNIQUE_1) -> TMEasy5/10
  InputFromCTRL/4(AddLatRoadSlope[-]___UNIQUE_1) -> TMEasy5/11
  InputFromCTRL/5(LocalRoadSysSwitch[0;1]___UNIQUE_1) -> TMEasy5/12
  TMEasy5/27 -> Demux2/1
  TMEasy5/1 -> TireOutput/1(ContactPointPos_wrt_WheelCenter(WorldSys)[m]___UNIQUE_1)
  TMEasy5/2 -> TireOutput/2(CamberAng(ContactSys)[rad]___UNIQUE_1)
  TMEasy5/3 -> TireOutput/3(TireDefl[m]___UNIQUE_1)
  TMEasy5/4 -> TireOutput/4(TireDeflSpd[m/s]___UNIQUE_1)
  TMEasy5/5 -> TireOutput/5(LongSpd(ContactSys)[m/s]___UNIQUE_1)
  TMEasy5/6 -> TireOutput/6(LatSpd(ContactSys)[m/s]___UNIQUE_1)
  TMEasy5/7 -> TireOutput/7(BoreSpd(ContactSys)[rad/s]___UNIQUE_1)
  TMEasy5/8 -> TireOutput/8(LongFrcLeverArm_wrt_WheelRotAxis[m]___UNIQUE_1)
  TMEasy5/9 -> TireOutput/9(LongUnitVector(WorldSys)[-]___UNIQUE_1)
  TMEasy5/10 -> TireOutput/10(LatUnitVector(WorldSys)[-]___UNIQUE_1)
  TMEasy5/11 -> TireOutput/11(RoadNormalVector(WorldSys)[-]___UNIQUE_1)
  TMEasy5/12 -> TireOutput/12(RoadType[-]___UNIQUE_1)
  TMEasy5/13 -> TireOutput/13(RoadFrictionScalingCoeff[-]___UNIQUE_1)
  TMEasy5/14 -> TireOutput/14(ContactPointPos(WorldSys)[m]___UNIQUE_1)
  TMEasy5/15 -> TireOutput/15(WheelCenterFrc(VehSys)[N]___UNIQUE_1)
  TMEasy5/16 -> TireOutput/16(WheelCenterTrq(VehSys)[Nm]___UNIQUE_1)
  TMEasy5/17 -> TireOutput/17(CircumferentialTrq_wrt_WheelRotAxis[Nm]___UNIQUE_1)
  TMEasy5/18 -> TireOutput/18(MaxRollResistTrq[Nm]___UNIQUE_1)
  TMEasy5/19 -> TireOutput/19(LatDefl(ContactSys)[m]___UNIQUE_1)
  TMEasy5/20 -> TireOutput/20(VertStiff[N/m]___UNIQUE_1)
  TMEasy5/21 -> TireOutput/21(UnloadedRadius[m]___UNIQUE_1)
  TMEasy5/22 -> TireOutput/22(RimRadius[m]___UNIQUE_1)
  TMEasy5/23 -> TireOutput/23(Width[m]___UNIQUE_1)
  TMEasy5/24 -> TireOutput/24(ContactPointFrc(ContactSys)[N]___UNIQUE_1)
  TMEasy5/25 -> TireOutput/25(CorneringStiff[N]___UNIQUE_1)
  TMEasy5/26 -> TireOutput/26(DynamicRadius[m]___UNIQUE_1)
  TMEasy5/28 -> TireOutput/32(SelfAligningTrq[Nm]___UNIQUE_1)
  TMEasy5/29 -> TireOutput/33(RollResistTrq[Nm]___UNIQUE_1)
  TMEasy5/30 -> TireOutput/34(TippingTrq[Nm]___UNIQUE_1)
  TMEasy5/31 -> TireOutput/35(BoreTrq[Nm]___UNIQUE_1)
  TMEasy5/32 -> Demux1/1
  TMEasy5/33 -> Demux3/1
  TMEasy5/34 -> TireOutput/50(BoreRadius[m]___UNIQUE_1)
  TMEasy5/35 -> TireOutput/51(TireRotSpd[rad/s]___UNIQUE_1)
  TMEasy5/36 -> TireOutput/52(CamberFrc[N]___UNIQUE_1)
  Demux4/1 -> TireOutput/53(LongRelaxationTime[s]___UNIQUE_1)
  Demux4/2 -> TireOutput/54(LatRelaxationTime[s]___UNIQUE_1)
  Demux4/3 -> TireOutput/55(TorsionalRelaxationTime[s]___UNIQUE_1)
  Demux5/1 -> TireOutput/56(LongRelaxationLength[m]___UNIQUE_1)
  Demux5/2 -> TireOutput/57(LatRelaxationLength[m]___UNIQUE_1)
  Demux5/3 -> TireOutput/58(TorsionalRelaxationAngle[rad]___UNIQUE_1)
  TMEasy5/37 -> Demux4/1
  TMEasy5/38 -> Demux5/1
  TMEasy5/39 -> TireOutput/59(ContactPointTrq(ContactSys)[Nm]___UNIQUE_1)
  TMEasy5/40 -> TireOutput/60(ContactPatchLength[m]___UNIQUE_1)
  TMEasy5/41 -> TireOutput/61(ContactPatchWidth[m]___UNIQUE_1)
  TMEasy5/42 -> TireOutput/62(LocalContactPoints(WorldSys)[m]___UNIQUE_1)
  TMEasy5/43 -> TireOutput/63(NumberOfLocalContactPoints[-]___UNIQUE_1)
